simulink model "helicopter_integral"  (Simulink 7.9)
settings: Solver=ode1  StartTime=0.0  StopTime=inf  FixedStep=0.002  RelTol=1e-3
values from neighbouring files (symbols this model uses):
  CMD_ELEV_POS_LIMIT_LOWER = elev_0*180/pi    (= -27.5)    [setup_lab_heli_3d_skeleton.m]
  CMD_ELEV_POS_LIMIT_UPPER = -CMD_ELEV_POS_LIMIT_LOWER    (= 27.5)    [setup_lab_heli_3d_skeleton.m]
  CMD_RATE_LIMIT = 45.0 * pi / 180    (= 0.785398163397)    [setup_lab_heli_3d_skeleton.m]
  elev_0 = -27.5*pi/180    (= -0.479965544298)    [setup_lab_heli_3d_skeleton.m]
  K_AMP = 5    [setup_lab_heli_3d_skeleton.m]
  K_JOYSTICK_X = 40.0    (= 40)    [setup_lab_heli_3d_skeleton.m]
  K_JOYSTICK_Y = 45.0    (= 45)    [setup_lab_heli_3d_skeleton.m]
  Ki = 0.1    [setup_lab_heli_3d_skeleton.m]
  Kr = 1    [setup_lab_heli_3d_skeleton.m]
  VMAX_AMP = 24    [setup_lab_heli_3d_skeleton.m]
  VMAX_DAC = 10    [setup_lab_heli_3d_skeleton.m]
  Vo = -1/2*g*(-m_w*Lw + m_f*La + m_b*La ) / (La*Kf)    [setup_lab_heli_3d_skeleton.m]
undefined symbols (not defined in the file or in its folder): A, B, C, CMD_TRAVEL_POS_LIMIT_LOWER, CMD_TRAVEL_POS_LIMIT_UPPER, HIL, K, K_EC_E, K_EC_P, K_EC_T, qc_get_step_size
libraries: quarc_library x5, simulink x2, simulink_extras x2
settings Model: Creator=MLevis  LastModifiedBy=s4291502  SimulationMode=external  ExtModeTrigDuration=10000
settings SolverCC: PositivePriorityOrder=on
settings OptimizationCC: InitFltsAndDblsToZero=on
settings DebuggingCC: SaveWithParameterizedLinksMsg=none  FcnCallInpInsideContextMsg=Use local settings  StrictBusMsg=Warning
settings RTWCC: SystemTargetFile=quarc_win64.tlc  TemplateMakefile=quarc_default_tmf  Description=QUARC Win64 Target  ProcessScript=quarc_win64_make_rtw_hook
settings STFCustomTargetCC: TargetPreCompLibLocation=C:\PROGRA~3\QUARC\lib\2012a\win64\release  CodeReplacementLibrary=ANSI_C  GeneratePreprocessorConditionals=Disable all  CombineOutputUpdateFcns=on  GRTInterface=off  SystemTargetFile=quarc_win64.tlc
settings GRTTargetCC: TargetPreCompLibLocation=C:\PROGRA~3\QUARC\lib\2012a\win64\release  ParMdlRefBuildCompliant=off  CompOptLevelCompliant=off  ConcurrentExecutionCompliant=off  MatFileLogging=off  ExtMode=on  ExtModeMexFile=quarc_comm

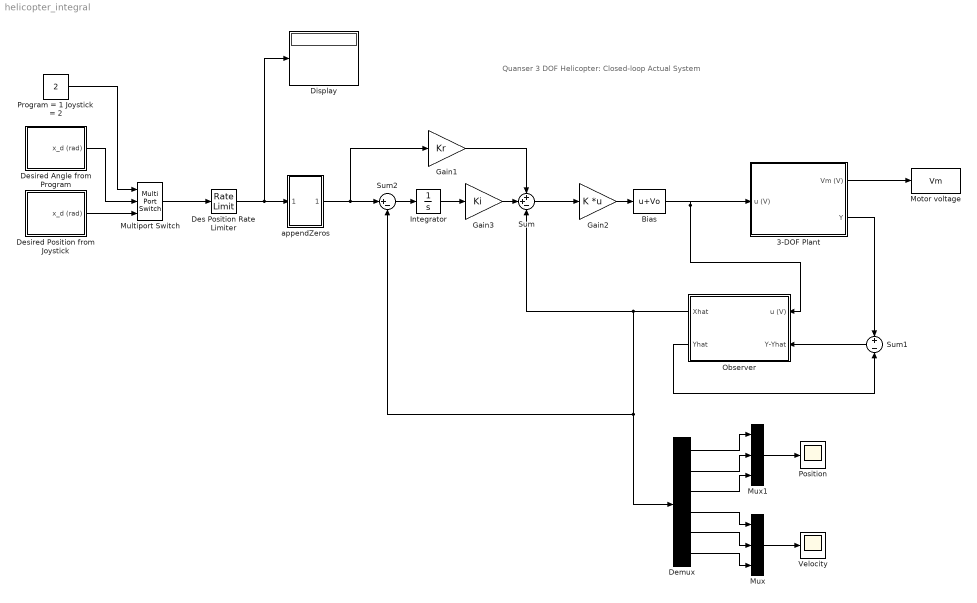
== system helicopter_integral ==
  note: Quanser 3 DOF Helicopter:
      | Closed-loop Actual System
  3-DOF Plant : Subsystem
  Bias : Bias  Bias=Vo
  Demux : Demux  Outputs=6
  Des Position Rate Limiter : RateLimiter  RisingSlewLimit=CMD_RATE_LIMIT  FallingSlewLimit=-CMD_RATE_LIMIT  SampleTimeMode=inherited
  Desired Angle from Program : Subsystem
  Desired Position from Joystick : Subsystem
  Display : Display
  Gain1 : Gain  Gain=Kr
  Gain2 : Gain  Gain=K  Multiplication=Matrix(K*u)
  Gain3 : Gain  Gain=Ki
  Integrator : Integrator
  Motor voltage : ToWorkspace  VariableName=Vm  SampleTime=-1
  Multiport Switch : MultiPortSwitch  Inputs=2  zeroidx=off
  Mux : Mux  Inputs=3
  Mux1 : Mux  Inputs=3
  Observer : Subsystem  TreatAsAtomicUnit=on
      settings: MinAlgLoopOccurrences=on
  Position : Scope
  Program = 1 Joystick = 2 : Constant  Value=2
  Sum : Sum  Inputs=++-
  Sum1 : Sum  Inputs=+|-
  Sum2 : Sum  Inputs=|+-
  Velocity : Scope
      settings: SaveName=ScopeData2
  appendZeros : Subsystem
  wires:
  Program = 1 Joystick = 2/1 -> Multiport Switch/1
  Desired Position from Joystick/1(x_d (rad)) -> Multiport Switch/3
  Multiport Switch/1 -> Des Position Rate Limiter/1
  3-DOF Plant/1(Vm (V)) -> Motor voltage/1
  Des Position Rate Limiter/1 -> appendZeros/1(In1), Display/1
  Bias/1 -> Observer/1(u (V)), 3-DOF Plant/1(u (V))
  Desired Angle from Program/1(x_d (rad)) -> Multiport Switch/2
  Sum/1 -> Gain2/1
  Observer/1(Xhat) -> Demux/1, Sum2/2, Sum/3
  Observer/2(Yhat) -> Sum1/2
  Sum1/1 -> Observer/2(Y-Yhat)
  3-DOF Plant/2(Y) -> Sum1/1
  Mux1/1 -> Position/1
  Mux/1 -> Velocity/1
  Demux/1 -> Mux1/1
  Demux/6 -> Mux/3
  Demux/5 -> Mux/2
  Demux/2 -> Mux1/2
  Demux/4 -> Mux/1
  Demux/3 -> Mux1/3
  appendZeros/1(Out1) -> Sum2/1, Gain1/1
  Gain1/1 -> Sum/1
  Integrator/1 -> Gain3/1
  Sum2/1 -> Integrator/1
  Gain2/1 -> Bias/1
  Gain3/1 -> Sum/2

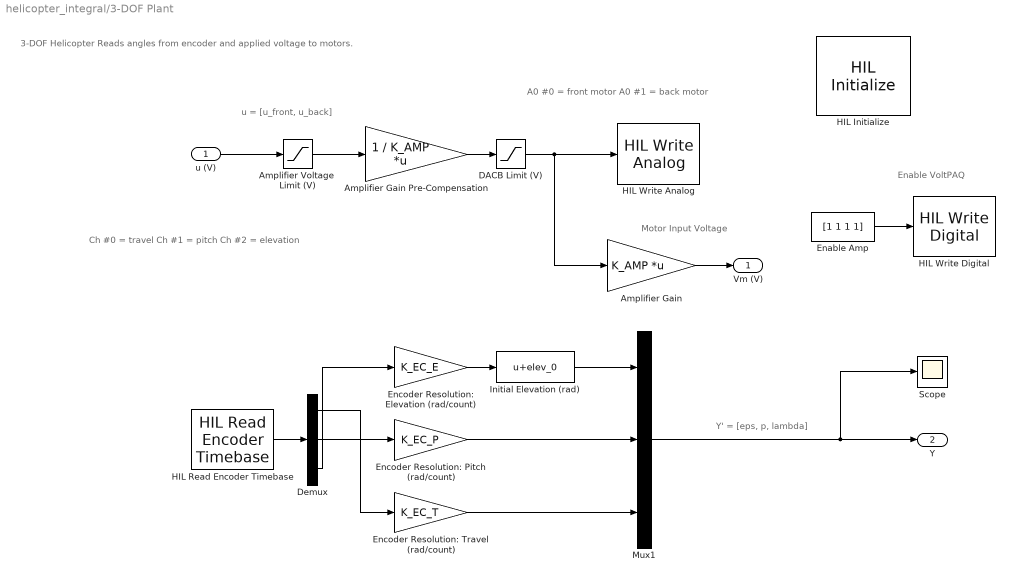
== system helicopter_integral/3-DOF Plant ==
  note: A0 #0 = front motor
      | A0 #1 = back motor
  note: u = [u_front, u_back]
  note: Motor Input Voltage
  note: 3-DOF Helicopter
      | Reads angles from encoder and applied voltage to motors.
  note: Ch #0 = travel
      | Ch #1 = pitch
      | Ch #2 = elevation
  note: Y' = [eps, p, lambda]
  note: Enable VoltPAQ
  u (V) : Inport
  Amplifier Gain : Gain  Gain=K_AMP  Multiplication=Matrix(K*u)  SaturateOnIntegerOverflow=on  OutDataTypeStr=Inherit: Same as input  ParamDataTypeStr=Inherit: Same as input
  Amplifier Gain Pre-Compensation : Gain  Gain=1 / K_AMP  Multiplication=Matrix(K*u)  SaturateOnIntegerOverflow=on  OutDataTypeStr=Inherit: Same as input  ParamDataTypeStr=Inherit: Same as input
  Amplifier Voltage  Limit (V) : Saturate  UpperLimit=VMAX_AMP  LowerLimit=-VMAX_AMP
  DACB Limit (V) : Saturate  UpperLimit=VMAX_DAC  LowerLimit=-VMAX_DAC
  Demux : Demux  Outputs=3
  Enable Amp : Constant  Value=[1 1 1 1]
  Encoder Resolution: Elevation (rad/count) : Gain  Gain=K_EC_E
  Encoder Resolution: Pitch (rad/count) : Gain  Gain=K_EC_P
  Encoder Resolution: Travel (rad/count) : Gain  Gain=K_EC_T
  HIL Initialize : quarc_library/Data Acquisition/Generic/Configuration/HIL Initialize  object_name=HIL-1  board_type=q4  board_number=0  exclusive=off  active=on  hardware_clocks=[0:1]  clock_modes=[0 0]  initial_clock_frequencies=[]  set_clock_params_at_start=on  set_clock_params_at_switch_in=off  set_clock_frequencies_at_start=off  set_clock_frequencies_at_switch_in=off  analog_input_channels=[0:3]  analog_input_maximums=10  analog_input_minimums=-10  set_analog_input_params_at_start=off  set_analog_input_params_at_switch_in=off  analog_output_channels=[0:3]  analog_output_maximums=[10]  analog_output_minimums=[-10]  initial_analog_outputs=[0]  final_analog_outputs=[0]  watchdog_analog_outputs=0  set_analog_output_params_at_start=on  set_analog_output_params_at_switch_in=off  set_analog_outputs_at_start=on  set_analog_outputs_at_switch_in=off  set_analog_outputs_at_terminate=on  set_analog_outputs_at_switch_out=off  set_analog_outputs_on_watchdog=off  digital_input_channels=[8:15]  digital_output_channels=[0:7]  digital_output_configuration=[]  initial_digital_outputs=[0]  final_digital_outputs=[0]  watchdog_digital_outputs=[2]  set_digital_output_params_at_start=off  set_digital_output_params_at_switch_in=off  set_digital_outputs_at_start=on  set_digital_outputs_at_switch_in=off  set_digital_outputs_at_terminate=on  set_digital_outputs_at_switch_out=off  set_digital_outputs_on_watchdog=off  encoder_channels=[0:3]  quadrature=[4]  encoder_filter_frequency=(1/60e-9)/1  initial_encoder_counts=[0]  set_encoder_params_at_start=on  set_encoder_params_at_switch_in=off  set_encoder_counts_at_start=on  set_encoder_counts_at_switch_in=off  pwm_channels=[]  pwm_modes=[0]  pwm_frequency=(1/60e-9)/1024  pwm_configuration=[]  pwm_alignment=[]  pwm_polarity=[]  pwm_leading_deadband=[]  pwm_trailing_deadband=[]  initial_pwm_outputs=[0]  final_pwm_outputs=[0]  watchdog_pwm_outputs=[]  set_pwm_params_at_start=on  set_pwm_params_at_switch_in=off  set_pwm_outputs_at_start=on  set_pwm_outputs_at_switch_in=off  set_pwm_outputs_at_terminate=on  set_pwm_outputs_at_switch_out=off  set_pwm_outputs_on_watchdog=off  other_output_channels=[]  initial_other_outputs=[]  final_other_outputs=[]  watchdog_other_outputs=[]  set_other_outputs_at_start=off  set_other_outputs_at_switch_in=off  set_other_outputs_at_terminate=off  set_other_outputs_at_switch_out=off  set_other_outputs_on_watchdog=off
  HIL Read Encoder Timebase : quarc_library/Data Acquisition/Generic/Timebases/HIL Read Encoder Timebase  object_name=HIL-1  clock=0  channels=[0:2]  samples_in_buffer=max(ceil(1/qc_get_step_size), 1)  active=on  vector_output=on  data_type_mode=Inherit via back propagation  data_type=double
  HIL Write Analog : quarc_library/Data Acquisition/Generic/Immediate I//O/HIL Write Analog  object_name=HIL-1  channels=[0,1]  sample_time=-1  active=off  vector_input=on
  HIL Write Digital : quarc_library/Data Acquisition/Generic/Immediate I//O/HIL Write Digital  object_name=HIL-1  channels=[0:3]  sample_time=-1  active=off  vector_input=on
  Initial Elevation (rad) : Bias  Bias=elev_0
  Mux1 : Mux  Inputs=3
  Scope : Scope
  Vm (V) : Outport
  Y : Outport  Port=2
  wires:
  HIL Read Encoder Timebase/1 -> Demux/1
  Mux1/1 -> Scope/1, Y/1
  Amplifier Gain Pre-Compensation/1 -> DACB Limit (V)/1
  Amplifier Voltage  Limit (V)/1 -> Amplifier Gain Pre-Compensation/1
  Amplifier Gain/1 -> Vm (V)/1
  u (V)/1 -> Amplifier Voltage  Limit (V)/1
  DACB Limit (V)/1 -> Amplifier Gain/1, HIL Write Analog/1
  Demux/3 -> Encoder Resolution: Elevation (rad/count)/1
  Demux/1 -> Encoder Resolution: Travel (rad/count)/1
  Demux/2 -> Encoder Resolution: Pitch (rad/count)/1
  Encoder Resolution: Elevation (rad/count)/1 -> Initial Elevation (rad)/1
  Encoder Resolution: Pitch (rad/count)/1 -> Mux1/2
  Encoder Resolution: Travel (rad/count)/1 -> Mux1/3
  Initial Elevation (rad)/1 -> Mux1/1
  Enable Amp/1 -> HIL Write Digital/1

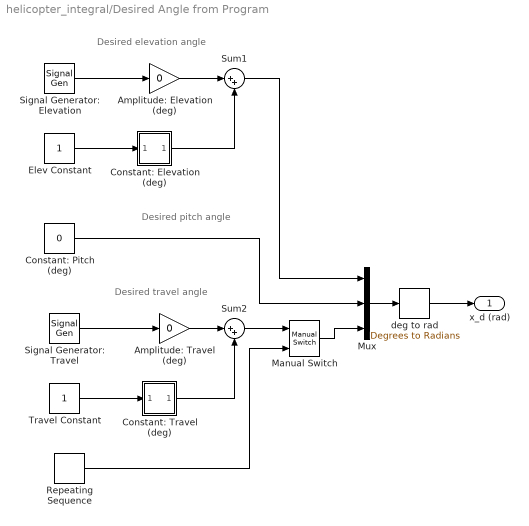
== system helicopter_integral/Desired Angle from Program ==
  note: Desired travel angle
  note: Desired elevation angle
  note: Desired pitch angle
  Amplitude: Elevation (deg) : Gain  Gain=0
  Amplitude: Travel (deg) : Gain  Gain=0
  Constant: Elevation (deg) : Subsystem  LoadFcn=slideg Load  StartFcn=slideg StartFcn  StopFcn=slideg StopFcn  mask(Slider Gain){low=-27.5, gain=-27.5, high=30}
      settings: CopyFcn=slideg Copy  DeleteFcn=slideg DeleteBlock  NameChangeFcn=slideg NameChange  OpenFcn=slideg Open  CloseFcn=slideg Close  ParentCloseFcn=slideg ParentClose
      mask Display: disp(gain)
  Constant: Pitch (deg) : Constant  Value=0
  Constant: Travel (deg) : Subsystem  LoadFcn=slideg Load  StartFcn=slideg StartFcn  StopFcn=slideg StopFcn  mask(Slider Gain){low=-90, gain=0, high=90}
      settings: CopyFcn=slideg Copy  DeleteFcn=slideg DeleteBlock  NameChangeFcn=slideg NameChange  OpenFcn=slideg Open  CloseFcn=slideg Close  ParentCloseFcn=slideg ParentClose
      mask Display: disp(gain)
  Elev Constant : Constant
  Manual Switch : simulink/Signal Routing/Manual Switch  sw=1  action=0  varsize=off
  Mux : Mux  Inputs=3
  Repeating Sequence : simulink/Sources/Repeating Sequence  rep_seq_t="[0  15 16  30  45  46 60 ]"  rep_seq_y="[0 0 30 30  30 0 0 ]"
  Signal Generator: Elevation : SignalGenerator  WaveForm=square  Frequency=0.04
  Signal Generator: Travel : SignalGenerator  WaveForm=square  Frequency=0.03
  Sum1 : Sum  Inputs=|++
  Sum2 : Sum  Inputs=|++
  Travel Constant : Constant
  deg to rad : simulink_extras/Transformations/Degrees to Radians
  x_d (rad) : Outport
  wires:
  deg to rad/1 -> x_d (rad)/1
  Signal Generator: Travel/1 -> Amplitude: Travel (deg)/1
  Amplitude: Travel (deg)/1 -> Sum2/1
  Travel Constant/1 -> Constant: Travel (deg)/1(In1)
  Sum1/1 -> Mux/1
  Signal Generator: Elevation/1 -> Amplitude: Elevation (deg)/1
  Amplitude: Elevation (deg)/1 -> Sum1/1
  Mux/1 -> deg to rad/1
  Constant: Pitch (deg)/1 -> Mux/2
  Elev Constant/1 -> Constant: Elevation (deg)/1(In1)
  Constant: Elevation (deg)/1(Out1) -> Sum1/2
  Constant: Travel (deg)/1(Out1) -> Sum2/2
  Sum2/1 -> Manual Switch/1
  Manual Switch/1 -> Mux/3
  Repeating Sequence/1 -> Manual Switch/2

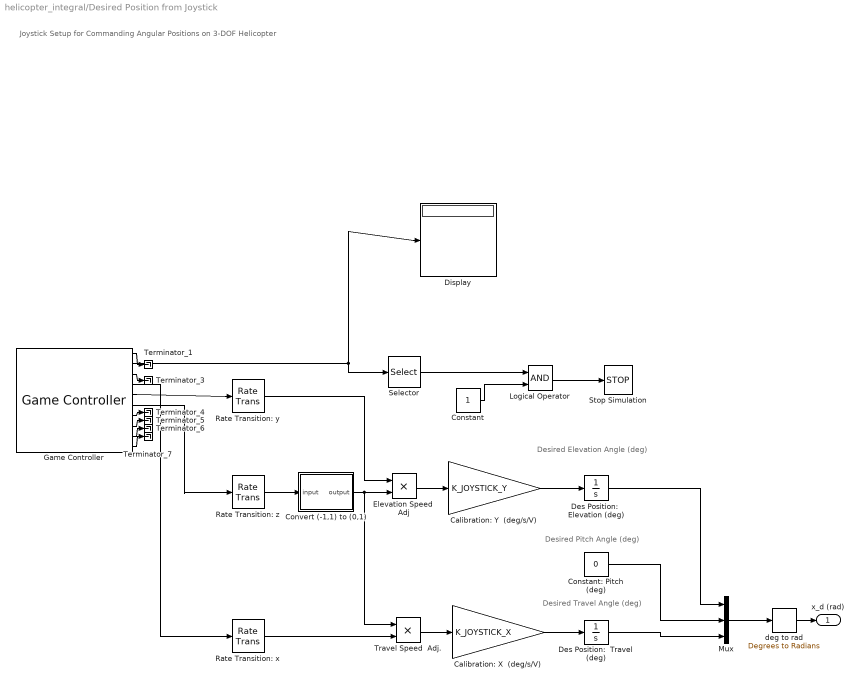
== system helicopter_integral/Desired Position from Joystick ==
  note: Desired Pitch Angle (deg)
  note: Desired Elevation Angle (deg)
  note: Desired Travel Angle (deg)
  note: Joystick Setup for Commanding Angular Positions on 3-DOF Helicopter
  Calibration: X  (deg/s/V) : Gain  Gain=K_JOYSTICK_X
  Calibration: Y  (deg/s/V) : Gain  Gain=K_JOYSTICK_Y
  Constant : Constant
  Constant: Pitch (deg) : Constant  Value=0
  Convert (-1,1) to (0,1) : Subsystem
  Des Position:  Elevation (deg) : Integrator  InitialCondition=elev_0*180/pi  LimitOutput=on  UpperSaturationLimit=CMD_ELEV_POS_LIMIT_UPPER  LowerSaturationLimit=CMD_ELEV_POS_LIMIT_LOWER
  Des Position:  Travel (deg) : Integrator  UpperSaturationLimit=CMD_TRAVEL_POS_LIMIT_UPPER  LowerSaturationLimit=CMD_TRAVEL_POS_LIMIT_LOWER
  Display : Display
  Elevation Speed  Adj : Product  RndMeth=Zero
  Game Controller : quarc_library/Devices/Peripherals/Target/Game Controller  controller=1  buffer_size=12  deadzone=[]  saturation=[]  sample_time=max(qc_get_step_size, 0.01)  auto_center=off  enabled=on
  Logical Operator : Logic  AllPortsSameDT=off  OutDataTypeStr=boolean
  Mux : Mux  Inputs=3
  Rate Transition: x : RateTransition
  Rate Transition: y : RateTransition
  Rate Transition: z : RateTransition
  Selector : Selector  InputPortWidth=32  IndexOptions=Index vector (dialog)  Indices=1  OutputSizes=1
  Stop Simulation : Stop
  Terminator_{1,3..7} (6 alike) : Terminator
  Travel Speed  Adj. : Product  RndMeth=Zero
  deg to rad : simulink_extras/Transformations/Degrees to Radians
  x_d (rad) : Outport
  wires:
  Des Position:  Elevation (deg)/1 -> Mux/1
  Mux/1 -> deg to rad/1
  deg to rad/1 -> x_d (rad)/1
  Calibration: X  (deg/s/V)/1 -> Des Position:  Travel (deg)/1
  Travel Speed  Adj./1 -> Calibration: X  (deg/s/V)/1
  Elevation Speed  Adj/1 -> Calibration: Y  (deg/s/V)/1
  Calibration: Y  (deg/s/V)/1 -> Des Position:  Elevation (deg)/1
  Convert (-1,1) to (0,1)/1(output) -> Travel Speed  Adj./1, Elevation Speed  Adj/2
  Rate Transition: z/1 -> Convert (-1,1) to (0,1)/1(input)
  Rate Transition: y/1 -> Elevation Speed  Adj/1
  Rate Transition: x/1 -> Travel Speed  Adj./2
  Game Controller/5 -> Rate Transition: y/1
  Game Controller/6 -> Rate Transition: z/1
  Game Controller/4 -> Rate Transition: x/1
  Game Controller/1 -> Terminator_1/1
  Game Controller/3 -> Terminator_3/1
  Game Controller/7 -> Terminator_4/1
  Game Controller/8 -> Terminator_5/1
  Game Controller/9 -> Terminator_6/1
  Game Controller/10 -> Terminator_7/1
  Des Position:  Travel (deg)/1 -> Mux/3
  Constant: Pitch (deg)/1 -> Mux/2
  Logical Operator/1 -> Stop Simulation/1
  Selector/1 -> Logical Operator/1
  Game Controller/2 -> Selector/1, Display/1
  Constant/1 -> Logical Operator/2

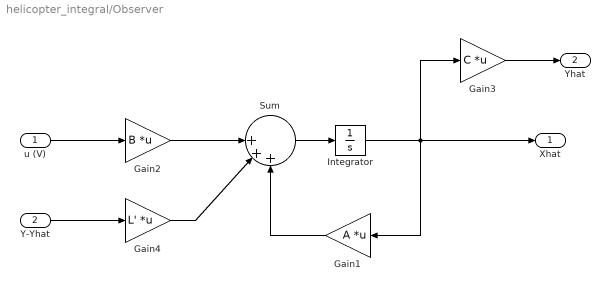
== system helicopter_integral/Observer ==
  u (V) : Inport
  Y-Yhat : Inport  Port=2
  Gain1 : Gain  Gain=A  Multiplication=Matrix(K*u)
  Gain2 : Gain  Gain=B  Multiplication=Matrix(K*u)
  Gain3 : Gain  Gain=C  Multiplication=Matrix(K*u)
  Gain4 : Gain  Gain=L'  Multiplication=Matrix(K*u)
  Integrator : Integrator
  Sum : Sum  Inputs=||+++
  Xhat : Outport
  Yhat : Outport  Port=2
  wires:
  u (V)/1 -> Gain2/1
  Gain2/1 -> Sum/1
  Y-Yhat/1 -> Gain4/1
  Gain1/1 -> Sum/3
  Sum/1 -> Integrator/1
  Integrator/1 -> Xhat/1, Gain1/1, Gain3/1
  Gain3/1 -> Yhat/1
  Gain4/1 -> Sum/2

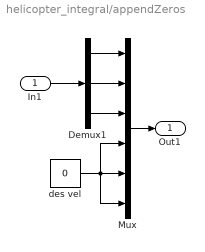
== system helicopter_integral/appendZeros ==
  In1 : Inport
  Demux1 : Demux  Outputs=3
  Mux : Mux  Inputs=6
  des vel : Constant  Value=0
  Out1 : Outport
  wires:
  Demux1/1 -> Mux/1
  Demux1/2 -> Mux/2
  Demux1/3 -> Mux/3
  des vel/1 -> Mux/5, Mux/4, Mux/6
  In1/1 -> Demux1/1
  Mux/1 -> Out1/1

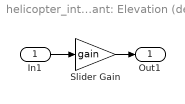
== system helicopter_integral/Desired Angle from Program/Constant: Elevation (deg) ==
  In1 : Inport
  Slider Gain : Gain  Gain=gain  SaturateOnIntegerOverflow=on  OutDataTypeStr=Inherit: Same as input  ParamDataTypeStr=Inherit: Same as input
  Out1 : Outport
  wires:
  In1/1 -> Slider Gain/1
  Slider Gain/1 -> Out1/1

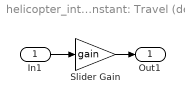
== system helicopter_integral/Desired Angle from Program/Constant: Travel (deg) ==
  In1 : Inport
  Slider Gain : Gain  Gain=gain  SaturateOnIntegerOverflow=on  OutDataTypeStr=Inherit: Same as input  ParamDataTypeStr=Inherit: Same as input
  Out1 : Outport
  wires:
  In1/1 -> Slider Gain/1
  Slider Gain/1 -> Out1/1

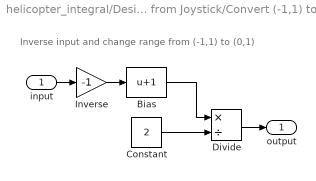
== system helicopter_integral/Desired Position from Joystick/Convert (-1,1) to (0,1) ==
  note: Inverse input and change range from (-1,1) to (0,1)
  input : Inport
  Bias : Bias  Bias=1
  Constant : Constant  Value=2
  Divide : Product  Inputs=*/
  Inverse : Gain  Gain=-1
  output : Outport
  wires:
  Constant/1 -> Divide/2
  Bias/1 -> Divide/1
  input/1 -> Inverse/1
  Divide/1 -> output/1
  Inverse/1 -> Bias/1
